simulink model "Xcvr_SSB_AM_2p5"  (Simulink 8.0)
settings: Solver=VariableStepDiscrete  SolverMode=SingleTasking  StartTime=0.0  StopTime=10  RelTol=1e-3
PreLoadFcn:
  | Fs=80e6;
  | 
  | phee=da_rom();
  | [phee_1,phee_2]=da_i2_rom();
  | 
  | Dcic=64;       % CIC decimation
  | Dfac=128;    % following DA filter decimation
  | N = 6;           %       (2^(N+1))=Dfac
  | Daudio=Dcic*Dfac;
  | Faudio=Fs/Daudio;
  | 
  | load info_filt_ssb_4
  | load Serial_Intfc_Stream_5
  | 
  | % AGC related
  | x=0.5:1/256:(1-1/256);
  | addr=(x-0.5)*256;
  | y=1./x;
values from neighbouring files (symbols this model uses):
  Serial_Interface = [0 0 0 0 0 0 0 0 0 0 0 0 ... (11390 elements, 2x5695)]    [Serial_Intfc_Stream_5.mat]
undefined symbols (not defined in the file or in its folder): get, sided, Two, xlipgetpartsetting
undefined symbols (not defined in the file): ssb_coef
libraries: xbsIndex_r4 x1305, dspsrcs4 x5, simulink x2, dspsigops x2, dspsnks4 x1
(part 5 of 11)

== system Xcvr_SSB_AM_2p5/TX Filters I=8192/Control ==
  Valid : Inport
  Ifac : Inport  Port=2
  AddSub : xbsIndex_r4/AddSub  mode=Addition  use_carryin=off  use_carryout=off  en=off  latency=0  precision=User Defined  arith_type=Unsigned  n_bits=4  bin_pt=0  quantization=Truncate  overflow=Wrap  dbl_ovrd=off  use_behavioral_HDL=off  hw_selection=Fabric  pipelined=off  use_rpm=on  block_type=addsub
      settings: block_version=9.2.00
  AddSub1 : xbsIndex_r4/AddSub  mode=Subtraction  use_carryin=off  use_carryout=off  en=off  latency=0  precision=User Defined  arith_type=Unsigned  n_bits=4  bin_pt=0  quantization=Truncate  overflow=Wrap  dbl_ovrd=off  use_behavioral_HDL=off  hw_selection=Fabric  pipelined=off  use_rpm=on  block_type=addsub
      settings: block_version=9.2.00
  Constant : xbsIndex_r4/Constant  const=0  gui_display_data_type=Fixed-point  arith_type=Unsigned  n_bits=7  bin_pt=0  preci_type=Single  exp_width=8  frac_width=24  explicit_period=off  period=1  equ=P=C  opselect=C  inp2=PCIN>>17  opr=+  inp1=P  carry=CIN  dbl_ovrd=off  block_type=constant
      settings: block_version=9.2.00
  Constant1 : xbsIndex_r4/Constant  const=32  gui_display_data_type=Fixed-point  arith_type=Unsigned  n_bits=7  bin_pt=0  preci_type=Single  exp_width=8  frac_width=24  explicit_period=off  period=1  equ=P=C  opselect=C  inp2=PCIN>>17  opr=+  inp1=P  carry=CIN  dbl_ovrd=off  block_type=constant
      settings: block_version=9.2.00
  Constant2 : xbsIndex_r4/Constant  const=64  gui_display_data_type=Fixed-point  arith_type=Unsigned  n_bits=7  bin_pt=0  preci_type=Single  exp_width=8  frac_width=24  explicit_period=off  period=1  equ=P=C  opselect=C  inp2=PCIN>>17  opr=+  inp1=P  carry=CIN  dbl_ovrd=off  block_type=constant
      settings: block_version=9.2.00
  Constant3 : xbsIndex_r4/Constant  const=96  gui_display_data_type=Fixed-point  arith_type=Unsigned  n_bits=7  bin_pt=0  preci_type=Single  exp_width=8  frac_width=24  explicit_period=off  period=1  equ=P=C  opselect=C  inp2=PCIN>>17  opr=+  inp1=P  carry=CIN  dbl_ovrd=off  block_type=constant
      settings: block_version=9.2.00
  Constant4 : xbsIndex_r4/Constant  const=0  gui_display_data_type=Fixed-point  arith_type=Unsigned  n_bits=7  bin_pt=0  preci_type=Single  exp_width=8  frac_width=24  explicit_period=off  period=1  equ=P=C  opselect=C  inp2=PCIN>>17  opr=+  inp1=P  carry=CIN  dbl_ovrd=off  block_type=constant
      settings: block_version=9.2.00
  Counter : xbsIndex_r4/Counter  cnt_type=Free Running  cnt_to=Inf  operation=Up  start_count=0  cnt_by_val=1  arith_type=Unsigned  n_bits=7  bin_pt=0  load_pin=off  rst=off  en=off  explicit_period=on  period=1/Fs  dbl_ovrd=off  use_behavioral_HDL=off  implementation=Fabric  use_rpm=off  block_type=counter
      settings: block_version=9.2.00
  Delay{,1..5} (6 alike) : xbsIndex_r4/Delay  rst=off  infoeditControl=Selection of Reset will increase slice count due to use of real FFs and instead of SRLs  en=off  latency=1  dbl_ovrd=off  reg_retiming=off  block_type=delay
      settings: block_version=12.1
  Logical : xbsIndex_r4/Logical  logical_function=OR  inputs=4  en=off  latency=0  precision=Full  arith_type=Unsigned  n_bits=16  bin_pt=0  align_bp=on  dbl_ovrd=off  block_type=logical
      settings: block_version=9.2.00
  Logical1 : xbsIndex_r4/Logical  logical_function=AND  inputs=3  en=off  latency=0  precision=Full  arith_type=Unsigned  n_bits=16  bin_pt=0  align_bp=on  dbl_ovrd=off  block_type=logical
      settings: block_version=9.2.00
  Reinterpret : xbsIndex_r4/Reinterpret  force_arith_type=on  arith_type=Unsigned  force_bin_pt=off  bin_pt=0  block_type=reinterpret
      settings: infoedit="Changes signal type without altering the binary representation.   You can changed the signal between signed and unsigned, and relocate the binary point.<P><P>Hardware notes: In hardware this block costs nothing.<P><P>Example:  Suppose the input is 6 bits wide, signed, with 2 fractional bits, and the output is forced to unsigned with 0 fractional bits.  Then an input of -2.0 (1110.00 in binary 2's complement) becomes an output of 56 (111000 in binary)."  block_version=9.2.00
  Reinterpret2 : xbsIndex_r4/Reinterpret  force_arith_type=on  arith_type=Unsigned  force_bin_pt=off  bin_pt=0  block_type=reinterpret
      settings: infoedit="Changes signal type without altering the binary representation.   You can changed the signal between signed and unsigned, and relocate the binary point.<P><P>Hardware notes: In hardware this block costs nothing.<P><P>Example:  Suppose the input is 6 bits wide, signed, with 2 fractional bits, and the output is forced to unsigned with 0 fractional bits.  Then an input of -2.0 (1110.00 in binary 2's complement) becomes an output of 56 (111000 in binary)."  block_version=9.2.00
  Relational{,1..3,5} (5 alike) : xbsIndex_r4/Relational  mode=a=b  en=off  latency=0  dbl_ovrd=off  block_type=relational
      settings: block_version=9.2.00
  Relational4 : xbsIndex_r4/Relational  mode=a>b  en=off  latency=0  dbl_ovrd=off  block_type=relational
      settings: block_version=9.2.00
  Shift : xbsIndex_r4/Shift  shift_dir=Left  shift_bits=3  en=off  latency=0  precision=User Defined  arith_type=Unsigned  n_bits=4  bin_pt=0  quantization=Truncate  overflow=Wrap  dbl_ovrd=off  block_type=shift
      settings: block_version=9.2.00
  Stage_Control : Subsystem
  bit_5 : xbsIndex_r4/Slice  nbits=1  boolean_output=on  mode=Lower Bit Location + Width  bit1=0  base1=MSB of Input  bit0=5  base0=LSB of Input  dbl_ovrd=off  block_type=slice
      settings: infoedit="Extracts a given range of bits from each input sample and presents it at the output.  The output type is ordinarily unsigned with binary point at zero, but can be Boolean when the slice is one bit wide.<P><P>Hardware notes: In hardware this block costs nothing."  block_version=9.2.00
  AB_Addr : Outport
  In_Sel : Outport  Port=2
  AB_Write : Outport  Port=3
  Real_Imag : Outport  Port=4
  AB_Sel : Outport  Port=5
  Start : Outport  Port=6
  SR_Addr : Outport  Port=7
  wires:
  AddSub/1 -> AddSub1/1, Delay2/1
  Shift/1 -> AddSub/1
  Logical1/1 -> Reinterpret/1, Delay4/1
  Valid/1 -> Logical1/3
  Reinterpret/1 -> AddSub1/2
  AddSub1/1 -> Delay3/1
  Relational5/1 -> Delay5/1
  Relational4/1 -> Logical1/2
  Constant/1 -> Relational/2
  Counter/1 -> Relational3/1, bit_5/1, Relational2/1, Relational1/1, Relational/1
  Relational/1 -> Logical/1
  Constant1/1 -> Relational1/2
  Constant2/1 -> Relational2/2
  Constant3/1 -> Relational3/2
  Relational1/1 -> Logical/2
  Relational2/1 -> Logical/3
  Relational3/1 -> Logical/4
  Logical/1 -> Delay/1
  bit_5/1 -> Reinterpret2/1, Delay1/1
  Constant4/1 -> Relational4/2
  Reinterpret2/1 -> Shift/1
  Ifac/1 -> Relational5/2
  Delay/1 -> Start/1
  Delay1/1 -> Real_Imag/1
  Delay2/1 -> SR_Addr/1
  Delay3/1 -> AB_Addr/1
  Delay4/1 -> AB_Write/1
  Delay5/1 -> In_Sel/1
  Stage_Control/3(AB_Sel) -> AB_Sel/1
  Stage_Control/1(Write_OK) -> Logical1/1
  Stage_Control/2(Filt_Stage) -> Relational4/1, AddSub/2, Relational5/1  "sr_addr"

== system Xcvr_SSB_AM_2p5/TX Filters I=8192/Fs_probe_1 ==
  In1 : Inport
  Probe : Probe  ProbeWidth=off  ProbeComplexSignal=off
  Product : Product  Inputs=/  RndMeth=Zero
  Selector : Selector  InputPortWidth=2  IndexOptions=Index vector (dialog)  Indices=1  OutputSizes=1
  Out1 : Outport
  wires:
  Selector/1 -> Product/1
  Probe/1 -> Selector/1
  In1/1 -> Probe/1
  Product/1 -> Out1/1

== system Xcvr_SSB_AM_2p5/TX Filters I=8192/Fs_probe_2 ==
  In1 : Inport
  Probe : Probe  ProbeWidth=off  ProbeComplexSignal=off
  Product : Product  Inputs=/  RndMeth=Zero
  Selector : Selector  InputPortWidth=2  IndexOptions=Index vector (dialog)  Indices=1  OutputSizes=1
  Out1 : Outport
  wires:
  Selector/1 -> Product/1
  Probe/1 -> Selector/1
  In1/1 -> Probe/1
  Product/1 -> Out1/1

== system Xcvr_SSB_AM_2p5/TX Filters I=8192/IO_Control ==
  Yn1 : Inport
  Yn2 : Inport  Port=2
  Real_In : Inport  Port=3
  Imag_In : Inport  Port=4
  AB_Addr : Inport  Port=5
  In_sel : Inport  Port=6
  Write : Inport  Port=7
  Real_Imag : Inport  Port=8
  AB_Sel : Inport  Port=9
  Mux : xbsIndex_r4/Mux  inputs=2  en=off  latency=0  precision=Full  arith_type=Unsigned  n_bits=16  bin_pt=14  quantization=Truncate  overflow=Wrap  dbl_ovrd=off  block_type=mux
      settings: block_version=9.2.00
  Mux1 : xbsIndex_r4/Mux  inputs=2  en=off  latency=0  precision=Full  arith_type=Unsigned  n_bits=16  bin_pt=14  quantization=Truncate  overflow=Wrap  dbl_ovrd=off  block_type=mux
      settings: block_version=9.2.00
  Mux2 : xbsIndex_r4/Mux  inputs=2  en=off  latency=0  precision=Full  arith_type=Unsigned  n_bits=16  bin_pt=14  quantization=Truncate  overflow=Wrap  dbl_ovrd=off  block_type=mux
      settings: block_version=9.2.00
  Reinterpret : xbsIndex_r4/Reinterpret  force_arith_type=on  arith_type="Signed  (2's comp)"  force_bin_pt=on  bin_pt=0  block_type=reinterpret
      settings: infoedit="Changes signal type without altering the binary representation.   You can changed the signal between signed and unsigned, and relocate the binary point.<P><P>Hardware notes: In hardware this block costs nothing.<P><P>Example:  Suppose the input is 6 bits wide, signed, with 2 fractional bits, and the output is forced to unsigned with 0 fractional bits.  Then an input of -2.0 (1110.00 in binary 2's complement) becomes an output of 56 (111000 in binary)."  block_version=9.2.00
  Reinterpret1 : xbsIndex_r4/Reinterpret  force_arith_type=on  arith_type="Signed  (2's comp)"  force_bin_pt=on  bin_pt=0  block_type=reinterpret
      settings: infoedit="Changes signal type without altering the binary representation.   You can changed the signal between signed and unsigned, and relocate the binary point.<P><P>Hardware notes: In hardware this block costs nothing.<P><P>Example:  Suppose the input is 6 bits wide, signed, with 2 fractional bits, and the output is forced to unsigned with 0 fractional bits.  Then an input of -2.0 (1110.00 in binary 2's complement) becomes an output of 56 (111000 in binary)."  block_version=9.2.00
  Single Port RAM : xbsIndex_r4/Single Port RAM  depth=16  initVector=zeros(1,16)  distributed_mem=Distributed memory  write_mode=Read Before Write  rst=off  init_reg=0  en=off  latency=0  dbl_ovrd=off  optimize=Area  block_type=spram
      settings: block_version=9.2.00
  Single Port RAM1 : xbsIndex_r4/Single Port RAM  depth=16  initVector=zeros(1,16)  distributed_mem=Distributed memory  write_mode=Read Before Write  rst=off  init_reg=0  en=off  latency=0  dbl_ovrd=off  optimize=Area  block_type=spram
      settings: block_version=9.2.00
  Xout : Outport
  wires:
  Write/1 -> Single Port RAM/3, Single Port RAM1/3
  In_sel/1 -> Mux1/1
  Mux1/1 -> Xout/1
  AB_Sel/1 -> Mux/1
  AB_Addr/1 -> Single Port RAM/1, Single Port RAM1/1
  Real_In/1 -> Reinterpret/1
  Real_Imag/1 -> Mux2/1
  Mux/1 -> Mux1/2
  Mux2/1 -> Mux1/3
  Reinterpret1/1 -> Mux2/3
  Single Port RAM1/1 -> Mux/2
  Single Port RAM/1 -> Mux/3
  Yn2/1 -> Single Port RAM1/2
  Yn1/1 -> Single Port RAM/2
  Reinterpret/1 -> Mux2/2
  Imag_In/1 -> Reinterpret1/1

== system Xcvr_SSB_AM_2p5/TX Filters I=8192/Interp_Core ==
  note: Rate=Fs
  Xin : Inport
  Start : Inport  Port=2
  SR_Addr : Inport  Port=3
  RAM Based SR : Subsystem
  ROM/Accumulator : Subsystem
  Register1 : xbsIndex_r4/Register  init=0  rst=off  en=on  dbl_ovrd=off  block_type=register
      settings: block_version=9.2.00
  Register2 : xbsIndex_r4/Register  init=0  rst=off  en=on  dbl_ovrd=off  block_type=register
      settings: block_version=9.2.00
  SAD_1 : Subsystem
  SAD_2 : Subsystem
  SAD_3 : Subsystem
  SAD_4 : Subsystem
  SRA : Subsystem
  SR_Yn : Subsystem
  SR_Zn : Subsystem
  Timing/Control1 : Subsystem
  Y RAM : xbsIndex_r4/Single Port RAM  depth=16  initVector=zeros(1,16)  distributed_mem=Distributed memory  write_mode=Read Before Write  rst=off  init_reg=0  en=off  latency=0  dbl_ovrd=off  optimize=Area  block_type=spram
      settings: block_version=9.2.00
  Z RAM : xbsIndex_r4/Single Port RAM  depth=16  initVector=zeros(1,16)  distributed_mem=Distributed memory  write_mode=Read Before Write  rst=off  init_reg=0  en=off  latency=0  dbl_ovrd=off  optimize=Area  block_type=spram
      settings: block_version=9.2.00
  Yn1_out : Outport
  Yn2_out : Outport  Port=2
  Valid : Outport  Port=3
  wires:
  SRA/1(Ser_Out) -> RAM Based SR/1(Xn_In)  "Xn"
  ROM/Accumulator/1(Yn) -> Register2/1
  Xin/1 -> SRA/1(Par_In)  "xn"
  SR_Yn/1(Ser_Out) -> RAM Based SR/2(Yn_in)
  SR_Zn/1(Ser_Out) -> RAM Based SR/3(Zn_in)
  RAM Based SR/1(Xn) -> SAD_1/1(A), SAD_3/1(A)
  RAM Based SR/5(Xn-4) -> SAD_1/2(B)
  SAD_1/1(Sum) -> ROM/Accumulator/1(Xn + Xn-4)
  RAM Based SR/2(Xn-1) -> SAD_2/1(A), SAD_4/1(A)
  RAM Based SR/4(Xn-3) -> SAD_2/2(B), SAD_3/2(B)
  SAD_2/1(Sum) -> ROM/Accumulator/2("Xn-1+ Xn-3 ")
  RAM Based SR/3(Xn-2) -> ROM/Accumulator/3(Xn-2), SAD_4/2(B)
  RAM Based SR/6(Yn-1) -> ROM/Accumulator/4(Yn-1)
  RAM Based SR/7(Yn-2) -> ROM/Accumulator/5(Yn-2)
  SAD_3/1(Sum) -> ROM/Accumulator/6(Xn+Xn-3)
  SAD_4/1(Sum) -> ROM/Accumulator/7(Xn-1+Xn-2)
  RAM Based SR/8(Zn-1) -> ROM/Accumulator/8(Zn-1)
  RAM Based SR/9(Zn-2) -> ROM/Accumulator/9(Zn-2)
  ROM/Accumulator/2(Zn) -> Register1/1
  Register2/1 -> Yn1_out/1, Y RAM/2
  Register1/1 -> Yn2_out/1, Z RAM/2
  Timing/Control1/2(Run) -> SRA/2(Shift), SR_Yn/2(Shift), SR_Zn/2(Shift)
  Timing/Control1/3(Clear_Adder) -> SAD_3/3(Clear), SAD_4/3(Clear), SAD_2/3(Clear), SAD_1/3(Clear)
  Timing/Control1/4(Round) -> ROM/Accumulator/10(Round)
  Timing/Control1/5(Clear_Acc) -> ROM/Accumulator/11(Clear Acc)
  Timing/Control1/6(Subtract) -> ROM/Accumulator/12(Subtract)
  Timing/Control1/7(Strobe) -> Register1/2, Register2/2
  SR_Addr/1 -> Z RAM/1, Y RAM/1, RAM Based SR/4(Addr)
  Start/1 -> Timing/Control1/1(Start)
  Timing/Control1/8(Valid) -> Valid/1, Z RAM/3, Y RAM/3
  Y RAM/1 -> SR_Yn/1(Par_In)
  Z RAM/1 -> SR_Zn/1(Par_In)
  Timing/Control1/1(SR Enable) -> RAM Based SR/5(En)
  Timing/Control1/9(Extend_Sign) -> RAM Based SR/6(Extend_Sign)

== system Xcvr_SSB_AM_2p5/Up/Down LO and Mixers/DDS_LO ==
  note: Changed to
      | Copy Samples
  Tx_Rx_Delayed : Inport
  RX_Write : Inport  Port=2
  TX_Write : Inport  Port=3
  Data : Inport  Port=4
  Delay : xbsIndex_r4/Delay  rst=off  infoeditControl=Selection of Reset will increase slice count due to use of real FFs and instead of SRLs  en=off  latency=1  dbl_ovrd=off  reg_retiming=off  block_type=delay
      settings: block_version=12.1
  Delay1 : xbsIndex_r4/Delay  rst=off  infoeditControl=Selection of Reset will increase slice count due to use of real FFs and instead of SRLs  en=off  latency=1  dbl_ovrd=off  reg_retiming=off  block_type=delay
      settings: block_version=12.1
  "LO_DDS Compiler 4.0 " : xbsIndex_r4/DDS Compiler 4.0   partspresent=Phase_Generator_and_SIN_COS_LUT  dds_clock_rate=Fs/1e6  channels=1  parameter_entry=System_Parameters  spurious_free_dynamic_range=86  frequency_resolution=Fs*2^-26 % was 2  noise_shaping=Taylor_Series_Corrected  phase_width=28  output_width=6  output_selection=Sine_and_Cosine  negative_sine=off  negative_cosine=off  amplitude_mode=Full_Range  memory_type=Auto  optimization_goal=Auto  dsp48_use=Minimal  latency_configuration=Auto  latency=6  has_phase_out=off  sclr_pin=off  clock_enable=off  rfd=off  rdy=on  channel_pin=off  explicit_period=on  period=1/Fs  phase_increment=Programmable  output_frequency1=0  output_frequency2=0  output_frequency3=0  output_frequency4=0  output_frequency5=0  output_frequency6=0  output_frequency7=0  output_frequency8=0  output_frequency9=0  output_frequency10=0  output_frequency11=0  output_frequency12=0  output_frequency13=0  output_frequency14=0  output_frequency15=0  output_frequency16=0  pinc1='0'  pinc2='0'  pinc3='0'  pinc4='0'  pinc5='0'  pinc6='0'  pinc7='0'  pinc8='0'  pinc9='0'  pinc10='0'  pinc11='0'  pinc12='0'  pinc13='0'  pinc14='0'  pinc15='0'  pinc16='0'  phase_offset=None  phase_offset_angles1=0  phase_offset_angles2=0  phase_offset_angles3=0  phase_offset_angles4=0  phase_offset_angles5=0  phase_offset_angles6=0  phase_offset_angles7=0  phase_offset_angles8=0  phase_offset_angles9=0  phase_offset_angles10=0  phase_offset_angles11=0  phase_offset_angles12=0  phase_offset_angles13=0  phase_offset_angles14=0  phase_offset_angles15=0  phase_offset_angles16=0  poff1='0'  poff2='0'  poff3='0'  poff4='0'  poff5='0'  poff6='0'  poff7='0'  poff8='0'  poff9='0'  poff10='0'  poff11='0'  poff12='0'  poff13='0'  poff14='0'  poff15='0'  poff16='0'  por_mode=false  gui_behaviour=Sysgen  ip_name=DDS Compiler  ip_version=4.0  dsptool_ready=true  wrapper_available=true  port_translation_map={ 'ce' => 'en', 'sclr' => 'rst' }  ipcore_xco_need_fpga_part=true  ipcore_fpga_part=xlipgetpartsetting(gcb, {'virtex4', 'xc4vsx35', '-10', 'ff668'})  ipcore_usecache=true  ipcore_useipmodelcache=true  ipcore_verbose=false  block_type=dds_compiler_v4_0
      settings: block_version=12.1
  Logical : xbsIndex_r4/Logical  logical_function=XOR  inputs=2  en=off  latency=0  precision=Full  arith_type=Unsigned  n_bits=16  bin_pt=0  align_bp=on  dbl_ovrd=off  block_type=logical
      settings: block_version=12.1
  Logical1 : xbsIndex_r4/Logical  logical_function=OR  inputs=2  en=off  latency=0  precision=Full  arith_type=Unsigned  n_bits=16  bin_pt=0  align_bp=on  dbl_ovrd=off  block_type=logical
      settings: block_version=12.1
  Mux : xbsIndex_r4/Mux  inputs=2  en=off  latency=0  precision=Full  arith_type=Unsigned  n_bits=16  bin_pt=14  quantization=Truncate  overflow=Wrap  dbl_ovrd=off  block_type=mux
      settings: block_version=12.1
  RX_Freq : xbsIndex_r4/Register  init=0  rst=off  en=on  dbl_ovrd=off  block_type=register
      settings: block_version=12.1
  Reinterpret : xbsIndex_r4/Reinterpret  force_arith_type=on  arith_type=Unsigned  force_bin_pt=on  bin_pt=26  block_type=reinterpret
      settings: infoedit="Changes signal type without altering the binary representation.   You can changed the signal between signed and unsigned, and relocate the binary point.<br><br>Hardware notes: In hardware this block costs nothing.<br><br>Example:  Suppose the input is 6 bits wide, signed, with 2 fractional bits, and the output is forced to unsigned with 0 fractional bits.  Then an input of -2.0 (1110.00 in binary 2's complement) becomes an output of 56 (111000 in binary)."  block_version=12.1
  TX_Freq : xbsIndex_r4/Register  init=0  rst=off  en=on  dbl_ovrd=off  block_type=register
      settings: block_version=12.1
  Up Sample : xbsIndex_r4/Up Sample  sample_ratio=8  copy_samples=on  en=off  latency=0  dbl_ovrd=off  block_type=usamp
      settings: block_version=9.2.00
  Up Sample1 : xbsIndex_r4/Up Sample  sample_ratio=8  copy_samples=on  en=off  latency=0  dbl_ovrd=off  block_type=usamp
      settings: block_version=9.2.00
  Out1 : Outport
  Out2 : Outport  Port=2
  Out3 : Outport  Port=3
  wires:
  Up Sample/1 -> "LO_DDS Compiler 4.0 "/2
  Up Sample1/1 -> "LO_DDS Compiler 4.0 "/1
  Reinterpret/1 -> Up Sample/1
  "LO_DDS Compiler 4.0 "/1 -> Out1/1
  "LO_DDS Compiler 4.0 "/2 -> Out2/1
  Data/1 -> RX_Freq/1, TX_Freq/1
  "LO_DDS Compiler 4.0 "/3 -> Out3/1
  RX_Write/1 -> Delay/1, RX_Freq/2
  TX_Write/1 -> TX_Freq/2
  RX_Freq/1 -> Mux/2
  Tx_Rx_Delayed/1 -> Mux/1, Delay1/1, Logical/1
  TX_Freq/1 -> Mux/3
  Mux/1 -> Reinterpret/1
  Delay1/1 -> Logical/2
  Logical/1 -> Logical1/2
  Delay/1 -> Logical1/1
  Logical1/1 -> Up Sample1/1

== system Xcvr_SSB_AM_2p5/Up/Down LO and Mixers/Delay allow T/R  Relay time. ==
  note: When going from T to R,
      | delay activating the ADC a bit more
      | to allow RFPA T/R relay to switch
  Tx_Rx_Delayed : Inport
  Delay : xbsIndex_r4/Delay  rst=off  infoeditControl=Selection of Reset will increase slice count due to use of real FFs and instead of SRLs  en=off  latency=1  dbl_ovrd=off  reg_retiming=off  block_type=delay
      settings: block_version=12.1
  Inverter1 : xbsIndex_r4/Inverter  en=off  latency=0  dbl_ovrd=off  block_type=inv
      settings: block_version=12.1
  Logical : xbsIndex_r4/Logical  logical_function=AND  inputs=2  en=off  latency=0  precision=Full  arith_type=Unsigned  n_bits=16  bin_pt=0  align_bp=on  dbl_ovrd=off  block_type=logical
      settings: block_version=12.1
  Logical3 : xbsIndex_r4/Logical  logical_function=OR  inputs=2  en=off  latency=0  precision=Full  arith_type=Unsigned  n_bits=16  bin_pt=0  align_bp=on  dbl_ovrd=off  block_type=logical
      settings: block_version=12.1
  N_Sample_One_Shot : Subsystem  mask{N=127}
      mask prompts: N "N=   (2<N<=255)"
  ADC_OFF : Outport
  wires:
  Tx_Rx_Delayed/1 -> Inverter1/1, Delay/1, Logical3/1
  Logical/1 -> N_Sample_One_Shot/1(In)  "Tx_to_Rx"
  N_Sample_One_Shot/1(Out) -> Logical3/2
  Inverter1/1 -> Logical/2
  Logical3/1 -> ADC_OFF/1
  Delay/1 -> Logical/1

== system Xcvr_SSB_AM_2p5/Up/Down LO and Mixers/OverLoad_Det ==
  In1 : Inport
  Constant : xbsIndex_r4/Constant  const=0  gui_display_data_type=Fixed-point  arith_type=Unsigned  n_bits=8  bin_pt=0  preci_type=Single  exp_width=8  frac_width=24  explicit_period=off  period=1  equ=P=C  opselect=C  inp2=PCIN>>17  opr=+  inp1=P  carry=CIN  dbl_ovrd=off  block_type=constant
      settings: block_version=9.2.00
  Counter : xbsIndex_r4/Counter  cnt_type=Free Running  cnt_to=Inf  operation=Up  start_count=0  cnt_by_val=1  arith_type=Unsigned  n_bits=8  bin_pt=0  load_pin=off  rst=off  en=off  explicit_period=on  period=8192/Fs  dbl_ovrd=off  use_behavioral_HDL=off  implementation=Fabric  use_rpm=off  block_type=counter
      settings: block_version=9.2.00
  Down Sample : xbsIndex_r4/Down Sample  sample_ratio=64  sample_phase="Last Value of Frame  (most efficient)"  en=off  latency=1  dbl_ovrd=off  block_type=dsamp
      settings: block_version=9.2.00
  Inverter{,1..5} (6 alike) : xbsIndex_r4/Inverter  en=off  latency=0  dbl_ovrd=off  block_type=inv
      settings: block_version=9.2.00
  Logical : xbsIndex_r4/Logical  logical_function=AND  inputs=6  en=off  latency=0  precision=Full  arith_type=Unsigned  n_bits=16  bin_pt=0  align_bp=on  dbl_ovrd=off  block_type=logical
      settings: block_version=9.2.00
  Logical1 : xbsIndex_r4/Logical  logical_function=AND  inputs=6  en=off  latency=0  precision=Full  arith_type=Unsigned  n_bits=16  bin_pt=0  align_bp=on  dbl_ovrd=off  block_type=logical
      settings: block_version=9.2.00
  Logical2 : xbsIndex_r4/Logical  logical_function=OR  inputs=2  en=off  latency=1  precision=Full  arith_type=Unsigned  n_bits=16  bin_pt=0  align_bp=on  dbl_ovrd=off  block_type=logical
      settings: block_version=9.2.00
  Logical3 : xbsIndex_r4/Logical  logical_function=OR  inputs=2  en=off  latency=0  precision=Full  arith_type=Unsigned  n_bits=16  bin_pt=0  align_bp=on  dbl_ovrd=off  block_type=logical
      settings: block_version=9.2.00
  Register : xbsIndex_r4/Register  init=0  rst=on  en=off  dbl_ovrd=off  block_type=register
      settings: block_version=9.2.00
  Relational : xbsIndex_r4/Relational  mode=a=b  en=off  latency=0  dbl_ovrd=off  block_type=relational
      settings: block_version=9.2.00
  Slice : xbsIndex_r4/Slice  nbits=1  boolean_output=on  mode=Upper Bit Location + Width  bit1=0  base1=MSB of Input  bit0=0  base0=LSB of Input  dbl_ovrd=off  block_type=slice
      settings: infoedit="Extracts a given range of bits from each input sample and presents it at the output.  The output type is ordinarily unsigned with binary point at zero, but can be Boolean when the slice is one bit wide.<P><P>Hardware notes: In hardware this block costs nothing."  block_version=9.2.00
  Slice1 : xbsIndex_r4/Slice  nbits=1  boolean_output=on  mode=Upper Bit Location + Width  bit1=-1  base1=MSB of Input  bit0=0  base0=LSB of Input  dbl_ovrd=off  block_type=slice
      settings: infoedit="Extracts a given range of bits from each input sample and presents it at the output.  The output type is ordinarily unsigned with binary point at zero, but can be Boolean when the slice is one bit wide.<P><P>Hardware notes: In hardware this block costs nothing."  block_version=9.2.00
  Slice2 : xbsIndex_r4/Slice  nbits=1  boolean_output=on  mode=Upper Bit Location + Width  bit1=-2  base1=MSB of Input  bit0=0  base0=LSB of Input  dbl_ovrd=off  block_type=slice
      settings: infoedit="Extracts a given range of bits from each input sample and presents it at the output.  The output type is ordinarily unsigned with binary point at zero, but can be Boolean when the slice is one bit wide.<P><P>Hardware notes: In hardware this block costs nothing."  block_version=9.2.00
  Slice3 : xbsIndex_r4/Slice  nbits=1  boolean_output=on  mode=Upper Bit Location + Width  bit1=-3  base1=MSB of Input  bit0=0  base0=LSB of Input  dbl_ovrd=off  block_type=slice
      settings: infoedit="Extracts a given range of bits from each input sample and presents it at the output.  The output type is ordinarily unsigned with binary point at zero, but can be Boolean when the slice is one bit wide.<P><P>Hardware notes: In hardware this block costs nothing."  block_version=9.2.00
  Slice4 : xbsIndex_r4/Slice  nbits=1  boolean_output=on  mode=Upper Bit Location + Width  bit1=-4  base1=MSB of Input  bit0=0  base0=LSB of Input  dbl_ovrd=off  block_type=slice
      settings: block_version=9.2.00
  Slice5 : xbsIndex_r4/Slice  nbits=1  boolean_output=on  mode=Upper Bit Location + Width  bit1=-5  base1=MSB of Input  bit0=0  base0=LSB of Input  dbl_ovrd=off  block_type=slice
      settings: block_version=9.2.00
  Out1 : Outport
  wires:
  Slice/1 -> Inverter/1, Logical1/1
  In1/1 -> Down Sample/1
  Inverter/1 -> Logical/1
  Slice1/1 -> Logical/2, Inverter1/1
  Slice2/1 -> Logical/3, Inverter2/1
  Slice3/1 -> Logical/4, Inverter3/1
  Inverter1/1 -> Logical1/2
  Inverter2/1 -> Logical1/3
  Inverter3/1 -> Logical1/4
  Logical1/1 -> Logical2/2
  Logical/1 -> Logical2/1
  Logical2/1 -> Logical3/1
  Logical3/1 -> Register/1
  Register/1 -> Logical3/2, Out1/1
  Relational/1 -> Register/2
  Counter/1 -> Relational/1
  Constant/1 -> Relational/2
  Down Sample/1 -> Slice/1, Slice1/1, Slice2/1, Slice3/1, Slice4/1, Slice5/1
  Slice4/1 -> Logical/5, Inverter4/1
  Slice5/1 -> Logical/6, Inverter5/1
  Inverter5/1 -> Logical1/6
  Inverter4/1 -> Logical1/5

== system Xcvr_SSB_AM_2p5/Audio_and_Mode_Control/AGC_and_More/AGC Xilinx ==
  note: In AM Mode, choose the largest Level be it audio or carrier.
  note: HI to force JCA_AGC
  note: 170312 was x0.5
  Data_In : Inport
  WR_AGC : Inport  Port=2
  Audio In : Inport  Port=3
  Tx_Rx_Delayed : Inport  Port=4
  AM_Mode : Inport  Port=5
  Carrier_Level : Inport  Port=6
  Tx_Rx : Inport  Port=7
  CW_nSSB : Inport  Port=8
  TX_Level : Inport  Port=9
  AGC_Reg : Subsystem
  Attack Filter : Subsystem  MinMaxOverflowLogging=MinMaxAndOverflow
  CMult : xbsIndex_r4/CMult  const=1.0  gui_display_data_type=Fixed-point  const_n_bits=3  const_bin_pt=2  float_type=Single  exp_bits=8  fraction_bits=24  en=off  latency=0  precision=User Defined  arith_type="Signed  (2's comp)"  n_bits=16  bin_pt=15  quantization=Truncate  overflow=Saturate  dbl_ovrd=off  use_behavioral_HDL=off  mem_type=Distributed RAM  pipeline=off  block_type=cmult
      settings: block_version=12.1
  Hang_Time : Subsystem  MinMaxOverflowLogging=MinMaxAndOverflow
  Inverter1 : xbsIndex_r4/Inverter  en=off  latency=0  dbl_ovrd=off  block_type=inv
      settings: block_version=9.2.00
  Leaky Peak Detector : Subsystem
  Logical : xbsIndex_r4/Logical  logical_function=AND  inputs=2  en=off  latency=0  precision=Full  arith_type=Unsigned  n_bits=16  bin_pt=0  align_bp=on  dbl_ovrd=off  block_type=logical
      settings: block_version=12.1
  Logical2 : xbsIndex_r4/Logical  logical_function=OR  inputs=2  en=off  latency=0  precision=Full  arith_type=Unsigned  n_bits=16  bin_pt=0  align_bp=on  dbl_ovrd=off  block_type=logical
      settings: block_version=9.2.00
  Mux4 : xbsIndex_r4/Mux  inputs=2  en=off  latency=0  precision=Full  arith_type=Unsigned  n_bits=26  bin_pt=26  quantization=Truncate  overflow=Wrap  dbl_ovrd=off  block_type=mux
      settings: block_version=9.2.00
  Mux7 : xbsIndex_r4/Mux  inputs=2  en=off  latency=0  precision=User Defined  arith_type=Unsigned  n_bits=24  bin_pt=23  quantization=Truncate  overflow=Wrap  dbl_ovrd=off  block_type=mux
      settings: block_version=9.2.00
  Relational3 : xbsIndex_r4/Relational  mode=a>b  en=off  latency=0  dbl_ovrd=off  block_type=relational
      settings: block_version=9.2.00
  S-Meter : Subsystem
  Sample Delay : Subsystem
  Sequential Divide : Subsystem
  Switch SW2 : xbsIndex_r4/Gateway In  gui_display_data_type=Fixed-point  arith_type=Boolean  n_bits=1  bin_pt=0  preci_type=Single  exp_width=8  frac_width=24  quantization="Round  (unbiased: +/- Inf)"  overflow=Saturate  period=1/Faudio  dbl_ovrd=off  timing_constraint=None  locs_specified=on  LOCs={'P93'}  UseAsADC=off  ADCChannel='1'  inherit_from_input=off  hdl_port=on  block_type=gatewayin
      settings: infoedit="Gateway in block.  Converts inputs of type Simulink integer, double and fixed point to  Xilinx fixed point type.<br><br>Hardware notes:  In hardware these blocks become top level input ports."  block_version=9.2.00
  Xabs : Subsystem
  Audio Out : Outport
  AGC_Level_TP : Outport  Port=2
  Shift_TP : Outport  Port=3
  AGC_Dig_TP : Outport  Port=4
  Smeter_PWM : Outport  Port=5
  wires:
  Xabs/1(Out1) -> Mux4/2, Mux7/2, Relational3/2
  Sequential Divide/2(Shift_TP) -> Shift_TP/1
  Tx_Rx_Delayed/1 -> Hang_Time/1(Tx_Rx_Delayed), Leaky Peak Detector/1(Tx_Rx_Delayed), Sequential Divide/1(Tx_Rx_Delayed), S-Meter/1(Tx_Rx_Delayed), Inverter1/1
  Leaky Peak Detector/1(Out1) -> AGC_Level_TP/1, Sequential Divide/3(Divisor), S-Meter/3(AGC_Divisor)
  Logical/1 -> Mux4/1
  AM_Mode/1 -> Logical/2
  Inverter1/1 -> Logical/1, Leaky Peak Detector/2(Rx_Tx_Delayed)
  Audio In/1 -> Xabs/1(In1), Sample Delay/1(Sample_In)
  Relational3/1 -> Mux7/1
  Mux7/1 -> Mux4/3
  Leaky Peak Detector/2(New_Max) -> Hang_Time/3(New_Max)
  Sample Delay/1(Out1) -> Sequential Divide/2(Dividend)
  WR_AGC/1 -> AGC_Reg/1(WR_AGC)
  Data_In/1 -> AGC_Reg/2(Data_in)
  AGC_Reg/3(Max_RX_Gain) -> Sequential Divide/4(Max_RX_Gain)
  Hang_Time/3(Hang_TP) -> AGC_Dig_TP/1
  Hang_Time/1(Trans_Reset) -> Sample Delay/3(Trans_Reset), Attack Filter/3(Trans_Reset)
  AGC_Reg/4(Max_Mic_Gain) -> Sequential Divide/5(Max_Mic_Gain)
  AGC_Reg/1(AGC_Hang) -> Hang_Time/2(Hang_load)
  Attack Filter/1(Out1) -> Leaky Peak Detector/3(Abs_In2)
  Hang_Time/2(Not_Hanging) -> Leaky Peak Detector/4(En)
  Mux4/1 -> Attack Filter/2(Abs_In1)
  AGC_Reg/2(AGC_Decay_Rate) -> Leaky Peak Detector/5(Rate)
  S-Meter/1(SMeter_PWM) -> Smeter_PWM/1
  Sequential Divide/3(Smeter) -> S-Meter/2(RX_Smeter)
  Tx_Rx/1 -> S-Meter/4(Tx_Rx)
  CW_nSSB/1 -> S-Meter/5(CW_nSSB)
  TX_Level/1 -> S-Meter/6(TX_Level)
  Switch SW2/1 -> Logical2/2
  AGC_Reg/5(JCA_AGC) -> Logical2/1
  Logical2/1 -> Sample Delay/2(JCA_AGC), Attack Filter/1(JCA_AGC)
  CMult/1 -> Audio Out/1
  Sequential Divide/1(Audio) -> CMult/1
  Carrier_Level/1 -> Relational3/1, Mux7/3

== system Xcvr_SSB_AM_2p5/Audio_and_Mode_Control/AGC_and_More/Over_Modulation_Detector ==
  note: If the AM_In upper 10 bits are zero
      |  then flag it as overmodulation.
  AM_Mode : Inport
  AM_In : Inport  Port=2
  Tx_Rx_Delayed : Inport  Port=3
  Constant1 : xbsIndex_r4/Constant  const=0  gui_display_data_type=Fixed-point  arith_type=Unsigned  n_bits=10  bin_pt=0  preci_type=Single  exp_width=8  frac_width=24  explicit_period=off  period=1  equ=P=C  opselect=C  inp2=PCIN>>17  opr=+  inp1=P  carry=CIN  dbl_ovrd=off  block_type=constant
      settings: block_version=12.1
  Logical1 : xbsIndex_r4/Logical  logical_function=AND  inputs=3  en=off  latency=0  precision=Full  arith_type=Unsigned  n_bits=16  bin_pt=0  align_bp=on  dbl_ovrd=off  block_type=logical
      settings: block_version=12.1
  Relational1 : xbsIndex_r4/Relational  mode=a=b  en=off  latency=1  dbl_ovrd=off  block_type=relational
      settings: block_version=12.1
  Slice upper  10 bits : xbsIndex_r4/Slice  nbits=10  boolean_output=off  mode=Upper Bit Location + Width  bit1=0  base1=MSB of Input  bit0=0  base0=LSB of Input  dbl_ovrd=off  block_type=slice
      settings: block_version=12.1
  OVER MODULATED : Outport
  wires:
  AM_In/1 -> Slice upper  10 bits/1
  Slice upper  10 bits/1 -> Relational1/1
  Constant1/1 -> Relational1/2
  Relational1/1 -> Logical1/1
  Logical1/1 -> OVER MODULATED/1
  AM_Mode/1 -> Logical1/2
  Tx_Rx_Delayed/1 -> Logical1/3

== system Xcvr_SSB_AM_2p5/Audio_and_Mode_Control/AGC_and_More/RX_Audio_Filter ==
  note: Added delay 7/31/2016
  note: [15 14 13 12 .... 3 2 1 0] [ 5 4 3 2 1 0] [ Bank_Sel] , [Reset], [WE] [Bypass]
  note: 16 Data 6 Address Bank Select Reset Write Enable Bypass
  note: 25 24 23 22 ....13 12 11 10 9 8 7 6 5 4 3 2 1 0
  note: To load WCS:
      | 1) Set Reset Bit then in a loop...
      | 2) With both Reset and WE set,
      | load 6 address and 16 Data bits. 64X for entire RAM.
      | 3) Lower both Reset and WE.
      | Yes one bit could do the job.
  Audio In : Inport
  Data_Fs/8 : Inport  Port=2
  WCS_Write : Inport  Port=3
  Tx_Rx_Delayed : Inport  Port=4
  Address_Slice : xbsIndex_r4/Slice  nbits=6  boolean_output=off  mode=Lower Bit Location + Width  bit1=-17  base1=LSB of Input  bit0=4  base0=LSB of Input  dbl_ovrd=off  block_type=slice
      settings: block_version=12.1
  Bank_Sel : xbsIndex_r4/Slice  nbits=1  boolean_output=on  mode=Lower Bit Location + Width  bit1=-17  base1=LSB of Input  bit0=3  base0=LSB of Input  dbl_ovrd=off  block_type=slice
      settings: block_version=12.1
  Bypass_Bit : xbsIndex_r4/Slice  nbits=1  boolean_output=on  mode=Lower Bit Location + Width  bit1=-17  base1=LSB of Input  bit0=0  base0=LSB of Input  dbl_ovrd=off  block_type=slice
      settings: block_version=12.1
  Data_Slice : xbsIndex_r4/Slice  nbits=16  boolean_output=off  mode=Lower Bit Location + Width  bit1=-17  base1=LSB of Input  bit0=10  base0=LSB of Input  dbl_ovrd=off  block_type=slice
      settings: block_version=12.1
  Down Sample : xbsIndex_r4/Down Sample  sample_ratio=1024/4  sample_phase="Last Value of Frame  (most efficient)"  en=off  latency=1  dbl_ovrd=off  block_type=dsamp
      settings: block_version=9.2.00
  Down Sample1 : xbsIndex_r4/Down Sample  sample_ratio=256  sample_phase=First Value of Frame  en=off  latency=0  dbl_ovrd=off  block_type=dsamp
      settings: block_version=9.2.00
  Down Sample3 : xbsIndex_r4/Down Sample  sample_ratio=4  sample_phase="Last Value of Frame  (most efficient)"  en=off  latency=1  dbl_ovrd=off  block_type=dsamp
      settings: block_version=9.2.00
  Logical : xbsIndex_r4/Logical  logical_function=OR  inputs=2  en=off  latency=0  precision=Full  arith_type=Unsigned  n_bits=16  bin_pt=0  align_bp=on  dbl_ovrd=off  block_type=logical
      settings: block_version=9.2.00
  Logical1 : xbsIndex_r4/Logical  logical_function=AND  inputs=2  en=off  latency=1  precision=Full  arith_type=Unsigned  n_bits=16  bin_pt=0  align_bp=on  dbl_ovrd=off  block_type=logical
      settings: block_version=12.1
  Register : xbsIndex_r4/Register  init=0  rst=off  en=on  dbl_ovrd=off  block_type=register
      settings: block_version=9.2.00
  Register2 : xbsIndex_r4/Register  init=0  rst=on  en=off  dbl_ovrd=off  block_type=register
      settings: block_version=9.2.00
  Reinterpret : xbsIndex_r4/Reinterpret  force_arith_type=on  arith_type="Signed  (2's comp)"  force_bin_pt=on  bin_pt=14  block_type=reinterpret
      settings: infoedit="Changes signal type without altering the binary representation.   You can changed the signal between signed and unsigned, and relocate the binary point.<br><br>Hardware notes: In hardware this block costs nothing.<br><br>Example:  Suppose the input is 6 bits wide, signed, with 2 fractional bits, and the output is forced to unsigned with 0 fractional bits.  Then an input of -2.0 (1110.00 in binary 2's complement) becomes an output of 56 (111000 in binary)."  block_version=12.1
  Reset_Bit : xbsIndex_r4/Slice  nbits=1  boolean_output=on  mode=Lower Bit Location + Width  bit1=-17  base1=LSB of Input  bit0=2  base0=LSB of Input  dbl_ovrd=off  block_type=slice
      settings: block_version=12.1
  Write_Enable : xbsIndex_r4/Slice  nbits=1  boolean_output=on  mode=Lower Bit Location + Width  bit1=-17  base1=LSB of Input  bit0=1  base0=LSB of Input  dbl_ovrd=off  block_type=slice
      settings: block_version=12.1
  n-tap MAC FIR Filter : Subsystem  mask(n-tap MAC FIR Filter){coef=[[-0.00818747392134573 -0.0210939731912657 0.00475497202799596 0.0100263011400189 -0.01704084314717 0.00592163002852389 0.0171246405970862 -0.0278547581464035 0.00727188844701682 0.0321996212084488 -0.0485233043393927 0.00812323371105136 0.0709878279041438 -0.111900071125327 0.00856366374654705 0.546493455780371 0.546493455780371 0.00856366374654705 -0.111900071125327 0.0709878279041438 0.00812323371105136 -0.0485233043393927 0.0321996212084488 0.00727188844701682 -0.0278547581464035 0.0171246405970862 0.00592163002852389 -0.01704084314717 0.0100263011400189 0.00475497202799596 -0.0210939731912657 -0.00818747392134573],zeros(1,32)], coef_n_bits=16, coef_bin_pt=14, smpl_n_bits=16, smpl_bin_pt=15, smpl_period=1/Faudio}
      mask prompts: coef "Coefficients"; coef_n_bits "Number of Bits per Coefficient"; coef_bin_pt "Binary Point for Coefficient"; smpl_n_bits "Number of Bits per Input Sample"; smpl_bin_pt "Binary Point for Input Samples"; smpl_period "Input Sample Period"
      mask help: MAC-based FIR filter with n coefficients.
      mask init:
      | dstr = sprintf('%d tap',length(coef));
      | 
      | [bg,fg] = xlcmap('XBlock',0);
      | iPos = get_param(gcb,'Position');
      | iWidth=iPos(3)-iPos(1); iHeight=iPos(4)-iPos(2);
      | iCx=iWidth/2;
      | iCy=iHeight/2;
      | [logoX, logoY] = xlogo(iPos);
      mask Help: eval('');xlDoc('-book','sysgen','-topic','n_tap_MAC_FIR_Filter');
  ByPass : Outport
  Audio_Out : Outport  Port=2
  wires:
  Audio In/1 -> n-tap MAC FIR Filter/2(din)
  n-tap MAC FIR Filter/1(dout) -> Audio_Out/1
  Reset_Bit/1 -> n-tap MAC FIR Filter/3(Reset)
  Write_Enable/1 -> Logical1/1
  Address_Slice/1 -> n-tap MAC FIR Filter/5(Coef_RAM_Addr)
  WCS_Write/1 -> Logical/2, Register/2
  Register/1 -> Down Sample/1
  Down Sample/1 -> Reset_Bit/1, Bypass_Bit/1, Write_Enable/1, Address_Slice/1, Bank_Sel/1, Data_Slice/1
  Data_Slice/1 -> Reinterpret/1
  Reinterpret/1 -> n-tap MAC FIR Filter/4(Coef)
  Down Sample1/1 -> Register2/2, Logical1/2  "we"
  Logical/1 -> Register2/1
  Register2/1 -> Down Sample1/1, Logical/1
  Logical1/1 -> n-tap MAC FIR Filter/7(we)
  Data_Fs/8/1 -> Register/1
  Bypass_Bit/1 -> Down Sample3/1
  Down Sample3/1 -> ByPass/1
  Tx_Rx_Delayed/1 -> n-tap MAC FIR Filter/1(Tx_Rx_Delayed)
  Bank_Sel/1 -> n-tap MAC FIR Filter/6(Bank_Sel)

== system Xcvr_SSB_AM_2p5/Audio_and_Mode_Control/AGC_and_More/RX_Audio_Select ==
  note: In Tx, use RX_EQ Filter for CW Sidetone, and
      | bypass Filters if AM or Bypass bit true.
  Tx_Rx_Delayed : Inport
  Sidetone_Filter_Audo : Inport  Port=2
  RXEQ_Bypass : Inport  Port=3
  RXEQ_Audio : Inport  Port=4
  RX_Audio_(unfiltered) : Inport  Port=5
  CW_nSSB : Inport  Port=6
  TX_Audio_Mon : Inport  Port=7
  Tx_Mon_EN : Inport  Port=8
  Tx_Rx_D40_&_CW : Inport  Port=9
  AM_Mode : Inport  Port=10
  Concat1 : xbsIndex_r4/Concat  num_inputs=2  dbl_ovrd=off  block_type=concat
      settings: block_version=12.1
  Inverter1 : xbsIndex_r4/Inverter  en=off  latency=0  dbl_ovrd=off  block_type=inv
      settings: block_version=9.2.00
  Inverter2 : xbsIndex_r4/Inverter  en=off  latency=0  dbl_ovrd=off  block_type=inv
      settings: block_version=9.2.00
  Logical1 : xbsIndex_r4/Logical  logical_function=OR  inputs=2  en=off  latency=0  precision=Full  arith_type=Unsigned  n_bits=16  bin_pt=0  align_bp=on  dbl_ovrd=off  block_type=logical
      settings: block_version=9.2.00
  Logical2 : xbsIndex_r4/Logical  logical_function=AND  inputs=3  en=off  latency=0  precision=Full  arith_type=Unsigned  n_bits=16  bin_pt=0  align_bp=on  dbl_ovrd=off  block_type=logical
      settings: block_version=9.2.00
  Logical3 : xbsIndex_r4/Logical  logical_function=AND  inputs=2  en=off  latency=0  precision=Full  arith_type=Unsigned  n_bits=16  bin_pt=0  align_bp=on  dbl_ovrd=off  block_type=logical
      settings: block_version=9.2.00
  Logical4 : xbsIndex_r4/Logical  logical_function=OR  inputs=2  en=off  latency=0  precision=Full  arith_type=Unsigned  n_bits=16  bin_pt=0  align_bp=on  dbl_ovrd=off  block_type=logical
      settings: block_version=9.2.00
  Mux2 : xbsIndex_r4/Mux  inputs=4  en=off  latency=1  precision=User Defined  arith_type="Signed  (2's comp)"  n_bits=16  bin_pt=15  quantization=Truncate  overflow=Wrap  dbl_ovrd=off  block_type=mux
      settings: block_version=9.2.00
  Mux6 : xbsIndex_r4/Mux  inputs=2  en=off  latency=0  precision=User Defined  arith_type="Signed  (2's comp)"  n_bits=16  bin_pt=15  quantization=Truncate  overflow=Wrap  dbl_ovrd=off  block_type=mux
      settings: block_version=9.2.00
  Switch SW1 : xbsIndex_r4/Gateway In  gui_display_data_type=Fixed-point  arith_type=Boolean  n_bits=1  bin_pt=0  preci_type=Single  exp_width=8  frac_width=24  quantization="Round  (unbiased: +/- Inf)"  overflow=Saturate  period=1/Faudio  dbl_ovrd=off  timing_constraint=None  locs_specified=on  LOCs={'P4'}  UseAsADC=off  ADCChannel='1'  inherit_from_input=off  hdl_port=on  block_type=gatewayin
      settings: infoedit="Gateway in block.  Converts inputs of type Simulink integer, double and fixed point to  Xilinx fixed point type.<br><br>Hardware notes:  In hardware these blocks become top level input ports."  block_version=9.2.00
  RX_Out : Outport
  wires:
  CW_nSSB/1 -> Inverter2/1
  Tx_Mon_EN/1 -> Logical1/2
  Logical1/1 -> Logical2/1
  Tx_Rx_Delayed/1 -> Logical2/3
  TX_Audio_Mon/1 -> Mux6/3
  Mux6/1 -> RX_Out/1
  Logical2/1 -> Mux6/1
  Concat1/1 -> Mux2/1
  Mux2/1 -> Mux6/2
  Logical3/1 -> Concat1/1
  RXEQ_Bypass/1 -> Logical3/1
  AM_Mode/1 -> Inverter1/1, Logical4/2
  RXEQ_Audio/1 -> Mux2/2
  Sidetone_Filter_Audo/1 -> Mux2/5, Mux2/3
  RX_Audio_(unfiltered)/1 -> Mux2/4
  Inverter1/1 -> Logical3/2
  Tx_Rx_D40_&_CW/1 -> Concat1/2
  Logical4/1 -> Logical2/2
  Inverter2/1 -> Logical4/1
  Switch SW1/1 -> Logical1/1

== system Xcvr_SSB_AM_2p5/Audio_and_Mode_Control/AGC_and_More/RX_Audio_to_Filters_Select ==
  note: CW & TX = sidetone,
      | otherwise TX = 0.
      | RX audio during RX
  Tx_Rx_Delayed : Inport
  CW_nSSB : Inport  Port=2
  Tx_Rx : Inport  Port=3
  Sidetone : Inport  Port=4
  RX_In : Inport  Port=5
  Concat2 : xbsIndex_r4/Concat  num_inputs=2  dbl_ovrd=off  block_type=concat
      settings: block_version=12.1
  Logical3 : xbsIndex_r4/Logical  logical_function=AND  inputs=2  en=off  latency=0  precision=Full  arith_type=Unsigned  n_bits=16  bin_pt=0  align_bp=on  dbl_ovrd=off  block_type=logical
      settings: block_version=9.2.00
  Mux7 : xbsIndex_r4/Mux  inputs=4  en=off  latency=1  precision=User Defined  arith_type="Signed  (2's comp)"  n_bits=16  bin_pt=15  quantization=Truncate  overflow=Wrap  dbl_ovrd=off  block_type=mux
      settings: block_version=9.2.00
  constant : xbsIndex_r4/Constant  const=0  gui_display_data_type=Fixed-point  arith_type=Signed (2's comp)  n_bits=16  bin_pt=15  preci_type=Single  exp_width=8  frac_width=24  explicit_period=on  period=8192/Fs  equ=P=C  opselect=C  inp2=PCIN>>17  opr=+  inp1=P  carry=CIN  dbl_ovrd=off  block_type=constant
      settings: block_version=9.2.00
  RX_Out : Outport
  wires:
  Tx_Rx/1 -> Logical3/1
  CW_nSSB/1 -> Logical3/2
  Logical3/1 -> Concat2/2
  Tx_Rx_Delayed/1 -> Concat2/1
  Concat2/1 -> Mux7/1
  constant/1 -> Mux7/4
  Sidetone/1 -> Mux7/5
  RX_In/1 -> Mux7/2, Mux7/3
  Mux7/1 -> RX_Out/1

== system Xcvr_SSB_AM_2p5/Audio_and_Mode_Control/AGC_and_More/TX Audio Select ==
  note: Audio for TX:
      | (0 during RX,
      | LFLO during CW TX,
      | Audio during voice TX)
  note: Two-Tone selection
      | supercedes all,
      | otherwise select
      | SSB (CW) or AM.
  note: Just add in DC carrier
      | level to create AM
  CW_Osc : Inport
  TX_Audio : Inport  Port=2
  AM_Mode : Inport  Port=3
  CW_nSSB : Inport  Port=4
  Tx_Rx : Inport  Port=5
  Two_Tone : Inport  Port=6
  TX_Carrier_Level : Inport  Port=7
  AM_Gen : xbsIndex_r4/AddSub  mode=Addition  use_carryin=off  use_carryout=off  en=off  latency=1  precision=User Defined  arith_type=Unsigned  n_bits=17  bin_pt=15  quantization="Round  (unbiased: +/- Inf)"  overflow=Saturate  dbl_ovrd=off  use_behavioral_HDL=off  hw_selection=Fabric  pipelined=off  use_rpm=on  block_type=addsub
      settings: block_version=9.2.00
  Concat : xbsIndex_r4/Concat  num_inputs=2  dbl_ovrd=off  block_type=concat
      settings: block_version=12.1
  Concat3 : xbsIndex_r4/Concat  num_inputs=2  dbl_ovrd=off  block_type=concat
      settings: block_version=12.1
  Mux1 : xbsIndex_r4/Mux  inputs=4  en=off  latency=1  precision=User Defined  arith_type="Signed  (2's comp)"  n_bits=16  bin_pt=15  quantization=Truncate  overflow=Wrap  dbl_ovrd=off  block_type=mux
      settings: block_version=9.2.00
  Mux4 : xbsIndex_r4/Mux  inputs=4  en=off  latency=1  precision=User Defined  arith_type="Signed  (2's comp)"  n_bits=16  bin_pt=15  quantization=Truncate  overflow=Wrap  dbl_ovrd=off  block_type=mux
      settings: block_version=9.2.00
  Two_Tone_Gen : Subsystem
  constant1 : xbsIndex_r4/Constant  const=0  gui_display_data_type=Fixed-point  arith_type=Signed (2's comp)  n_bits=16  bin_pt=15  preci_type=Single  exp_width=8  frac_width=24  explicit_period=on  period=8192/Fs  equ=P=C  opselect=C  inp2=PCIN>>17  opr=+  inp1=P  carry=CIN  dbl_ovrd=off  block_type=constant
      settings: block_version=9.2.00
  halve AM : xbsIndex_r4/CMult  const=0.5  gui_display_data_type=Fixed-point  const_n_bits=2  const_bin_pt=2  float_type=Single  exp_bits=8  fraction_bits=24  en=off  latency=0  precision=User Defined  arith_type="Signed  (2's comp)"  n_bits=16  bin_pt=15  quantization="Round  (unbiased: +/- Inf)"  overflow=Saturate  dbl_ovrd=off  use_behavioral_HDL=off  mem_type=Distributed RAM  pipeline=off  use_rpm=off  placement_style=Rectangular Shape  block_type=cmult
      settings: block_version=9.2.00
  TX_Out : Outport
  TX_AM_Out : Outport  Port=2
  wires:
  Tx_Rx/1 -> Concat/1
  CW_nSSB/1 -> Concat/2
  Concat/1 -> Mux4/1
  constant1/1 -> Mux4/3, Mux4/2
  TX_Audio/1 -> Mux4/4
  CW_Osc/1 -> Mux4/5
  Mux4/1 -> AM_Gen/1, Mux1/2
  TX_Carrier_Level/1 -> AM_Gen/2
  Two_Tone/1 -> Concat3/2
  AM_Mode/1 -> Concat3/1
  Concat3/1 -> Mux1/1
  halve AM/1 -> Mux1/4, TX_AM_Out/1
  AM_Gen/1 -> halve AM/1
  Two_Tone_Gen/1(Out1) -> Mux1/5, Mux1/3
  Mux1/1 -> TX_Out/1

== system Xcvr_SSB_AM_2p5/Audio_and_Mode_Control/AGC_and_More/Time_Share_MPY ==
  A : Inport
  X : Inport  Port=2
  B : Inport  Port=3
  Y : Inport  Port=4
  Mult2 : xbsIndex_r4/Mult  precision=User Defined  arith_type="Signed  (2's comp)"  n_bits=16  bin_pt=15  quantization=Truncate  overflow=Saturate  en=off  latency=2  dbl_ovrd=off  use_behavioral_HDL=off  opt=Area  use_embedded=on  optimum_pipeline=off  pipeline=on  use_rpm=on  placement_style=Triangular  block_type=mult
      settings: block_version=9.2.00
  Time Division Demultiplexer : xbsIndex_r4/Time Division Demultiplexer  frame_pattern=[1 1 ]  impl_style=Multiple Channel  vin=off  dbl_ovrd=off  explicit_period=off  period=1  block_type=tdd
      settings: infoedit=Samples presented at the input are selected and down-sampled according to the frame sampling pattern specified. The sampled input is presented either as a single or multiple channel at the output.  block_version=12.1
  Time Division Multiplexer : xbsIndex_r4/Time Division Multiplexer  inputs=2  vin=off  dbl_ovrd=off  explicit_period=off  period=1  block_type=tdm
      settings: infoedit="Multiple inputs are sampled and  presented serially at the output."  block_version=12.1
  Time Division Multiplexer1 : xbsIndex_r4/Time Division Multiplexer  inputs=2  vin=off  dbl_ovrd=off  explicit_period=off  period=1  block_type=tdm
      settings: infoedit="Multiple inputs are sampled and  presented serially at the output."  block_version=12.1
  A*X : Outport
  B*Y : Outport  Port=2
  wires:
  Time Division Multiplexer/1 -> Mult2/1
  Time Division Multiplexer1/1 -> Mult2/2
  Mult2/1 -> Time Division Demultiplexer/1
  A/1 -> Time Division Multiplexer/1
  B/1 -> Time Division Multiplexer/2
  X/1 -> Time Division Multiplexer1/1
  Y/1 -> Time Division Multiplexer1/2
  Time Division Demultiplexer/1 -> A*X/1
  Time Division Demultiplexer/2 -> B*Y/1
